simulink model "ThrusterTest"  (R2021a)
settings: Solver=FixedStepAuto  StartTime=0.0  StopTime=10  FixedStep=0.005  RelTol=1e-3  EnableMultiTasking=on
InitFcn:
  | loadThrusterData
  | loadSensorData
model workspace (MAT data in the model file):
  accelPhidget = [3707764736; 2; 1; 1; 1; 1]
  distPhidget1 = [3707764736; 2; 1; 1; 2; 2]
  distPhidget2 = [3707764736; 2; 1; 1; 3; 2]
  distPhidget3 = [3707764736; 2; 1; 1; 4; 2]
  distPhidget4 = [3707764736; 2; 1; 1; 5; 2]
  gyroPhidget = [3707764736; 2; 1; 1; 6; 3]
settings Model: EnablePacing=on  Creator=Andy  LastModifiedBy=Andy
settings SolverCC: AlgebraicLoopSolver=TrustRegion  PositivePriorityOrder=on
settings DataIOCC: SaveFormat=StructureWithTime  ReturnWorkspaceOutputs=off
settings OptimizationCC: EnhancedBackFolding=on  PassReuseOutputArgsAs=Individual arguments  ZeroExternalMemoryAtStartup=off  ZeroInternalMemoryAtStartup=off  MaxStackSize=64  OptimizeBlockOrder=speed  DifferentSizesBufferReuse=on  OptimizationCustomize=off  EfficientTunableParamExpr=on
settings DebuggingCC: ParameterTunabilityLossMsg=error  SFMachineParentedDataDiag=warning  ArithmeticOperatorsInVariantConditions=warning
settings HardwareCC: ProdBitPerPointer=32  ProdBitPerSizeT=32  ProdBitPerPtrDiffT=32  ProdLargestAtomicInteger=Long  ProdLargestAtomicFloat=Double  ProdWordSize=32  ProdHWDeviceType=ARM Compatible->ARM Cortex
settings ModelReferenceCC: ModelReferenceNumInstancesAllowed=Single
settings SFSimCC: MATLABDynamicMemAlloc=off  CustomCodeUndefinedFunction=UseInterfaceOnly  SimTargetLang=C++
settings RTWCC: SystemTargetFile=ert.tlc  HardwareBoard=Raspberry Pi  TLCOptions="-aInlineSetEventsForThisBaseRateFcn=TLC_TRUE -aSuppressMultiTaskScheduler=TLC_FALSE  -aRateBasedStepFcn=0"  GenCodeOnly=on  TemplateMakefile=ert_default_tmf  GenerateReport=on  Toolchain=GNU GCC Embedded Linux  BuildConfiguration=Faster Runs  IncludeHyperlinkInReport=on  LaunchReport=on  TargetLang=C++  GenerateTraceInfo=on  GenerateTraceReport=on  GenerateTraceReportSl=on  GenerateTraceReportSf=on  GenerateTraceReportEml=on
settings CodeAppCC: ForceParamTrailComments=on  IgnoreCustomStorageClasses=off  OperatorAnnotations=on  SimulinkDataObjDesc=on  SFDataObjDesc=on  InsertBlockDesc=on
settings ERTTargetCC: TargetLangStandard=C++03 (ISO)  MatFileLogging=on  CodeInterfacePackaging=C++ class  SupportVariableSizeSignals=on  MultiInstanceErrorCode=Warning  RootIOFormat=Structure reference

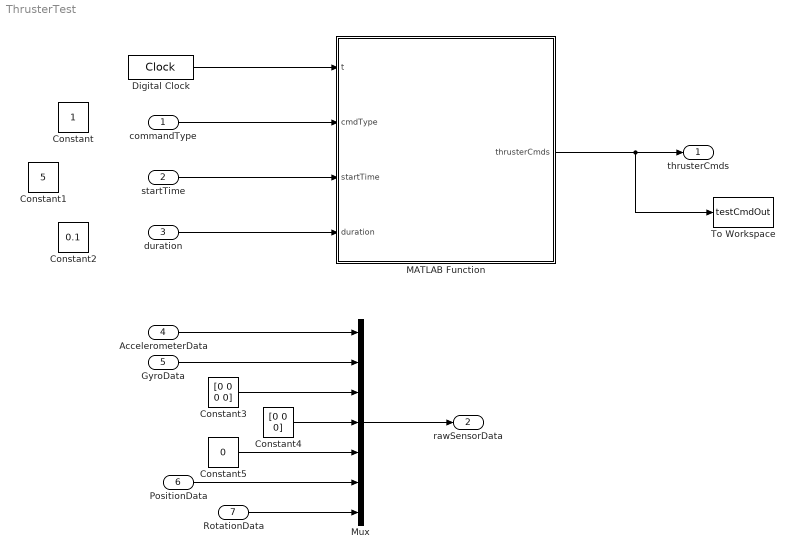
== system ThrusterTest ==
  commandType : Inport  OutDataTypeStr=int32
  startTime : Inport  Port=2
  duration : Inport  Port=3
  AccelerometerData : Inport  Port=4  OutDataTypeStr=double  PortDimensions=3
  GyroData : Inport  Port=5  OutDataTypeStr=double  PortDimensions=3
  PositionData : Inport  Port=6  OutDataTypeStr=double  PortDimensions=3
  RotationData : Inport  Port=7  OutDataTypeStr=double  PortDimensions=3
  Constant : Constant
  Constant1 : Constant  Value=5
  Constant2 : Constant  Value=0.1
  Constant3 : Constant  Value=[0 0 0 0]
  Constant4 : Constant  Value=[0 0 0]
  Constant5 : Constant  Value=0
  Digital Clock : DigitalClock  SampleTime=0.005
  MATLAB Function : MATLAB Function  TreatAsAtomicUnit=on
  Mux : Mux  Inputs=7
  To Workspace : ToWorkspace  VariableName=testCmdOut  SaveFormat=Timeseries  SampleTime=-1
  thrusterCmds : Outport  VectorParamsAs1DForOutWhenUnconnected=off
  rawSensorData : Outport  Port=2  VectorParamsAs1DForOutWhenUnconnected=off
  wires:
  MATLAB Function/1(thrusterCmds) -> To Workspace/1, thrusterCmds/1
  Digital Clock/1 -> MATLAB Function/1(t)
  commandType/1 -> MATLAB Function/2(cmdType)
  startTime/1 -> MATLAB Function/3(startTime)
  duration/1 -> MATLAB Function/4(duration)
  AccelerometerData/1 -> Mux/1
  GyroData/1 -> Mux/2
  Mux/1 -> rawSensorData/1
  Constant3/1 -> Mux/3
  Constant4/1 -> Mux/4
  Constant5/1 -> Mux/5
  PositionData/1 -> Mux/6
  RotationData/1 -> Mux/7

== matlab function ThrusterTest/MATLAB Function ==
  data: t input; thrusterCmds output; cmdType input; startTime input; duration input
function thrusterCmds = fcn(t,cmdType,startTime,duration)
%   Thruster Layout
%     3       2   
%    4         1
%
%
%    5         8       
%     6       7          ^
%                        | 
%  + X -->             + Y 

% cmdType firing axis
%    1 = +X Tran
%    2 = -X Tran
%    3 = +Y Tran
%    4 = -Y Tran
%    5 = +Z Rot 
%    6 = -Z Rot
%    11 = Thruster 1
%    12 = Thruster 2
%    13 = Thruster 3
%    14 = Thruster 4
%    15 = Thruster 5
%    16 = Thruster 6
%    17 = Thruster 7
%    18 = Thruster 8

% Default to zero each pass
thrusterCmds = zeros(1,8);
cmdNow = 0;

if t >= startTime
    if t < startTime+duration
        cmdNow = 1;
    end
end
   
if cmdNow == 1
    if cmdType == 1
        thrusterCmds(4) = 1;
        thrusterCmds(5) = 1;
    elseif cmdType == 2
        thrusterCmds(1) = 1;
        thrusterCmds(8) = 1;
    elseif cmdType == 3
        thrusterCmds(6) = 1;
        thrusterCmds(7) = 1;
    elseif cmdType == 4
        thrusterCmds(2) = 1;
        thrusterCmds(3) = 1;
    elseif cmdType == 5
        thrusterCmds(1) = 1;
        thrusterCmds(5) = 1;
    elseif cmdType == 6
        thrusterCmds(4) = 1;
        thrusterCmds(8) = 1;
    elseif cmdType >= 11 && cmdType <= 18
        thrusterCmds(cmdType-10) = 1;
    end
end
%     if mod(t,0.05) == 0
%         fprintf('Time is: %8.3f\n',t);
%     end
